simulink model "hydcyl4"  (Simulink 6.0)
settings: Solver=ode45  SolverMode=SingleTasking  StartTime=0.0  StopTime=0.1  FixedStep=0.001  RelTol=1e-5
PreLoadFcn:
  | load newhcd
values from neighbouring files (symbols this model uses):
  Ac = 0.001    [newhcd.mat]
  Beta = 700000000    [newhcd.mat]
  K = 50000    [newhcd.mat]
  Qmax = 0.005    [newhcd.mat]
libraries: hydlib x5
settings Model: Creator=The MathWorks Inc.  LastModifiedBy=batserve  ExtModeTrigMode=oneshot  ExtModeArmWhenConnect=off  ExtModeAutoUpdateStatusClock=off
settings DataIOCC: LimitDataPoints=off  SaveOutput=off  SaveState=on  SignalLoggingName=logsOut
settings OptimizationCC: BooleanDataType=off
settings DebuggingCC: AlgebraicLoopMsg=none  CheckExecutionContextPreStartOutputMsg=on  CheckExecutionContextRuntimeOutputMsg=on  SolverPrmCheckMsg=none  IntegerOverflowMsg=none
settings HardwareCC: TargetUnknown=on

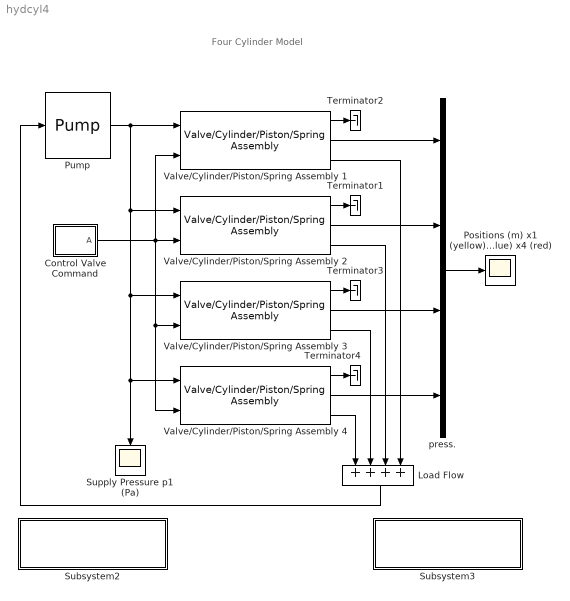
== system hydcyl4 ==
  note: Four Cylinder Model
  Control Valve Command : Subsystem  PropExecContextAcrossSSBoundary=on
      mask Type: Ramp
      mask Display: plot(0,0,100,100,[98,0],[96,0])
  Load Flow : Sum  Orientation=down  Inputs=++++  SaturateOnIntegerOverflow=on  InputSameDT=on
  Positions (m) x1 (yellow) x2 (purple) x3 (blue) x4 (red) : Scope
      settings: TickLabels=on  TimeRange=0.1  YMin=0  YMax=0.019  DataFormat=Array
  Pump : hydlib/Pump  t=[0 0.05 0.051 0.1]  Qpump=Qmax*[1 1 0.5 0.5]  p10=Qmax/C2/2  C2=C2
  Subsystem2 : Subsystem  PropExecContextAcrossSSBoundary=on
      settings: OpenFcn=sim(get_param(0,'CurrentSystem'),0.1)
      mask Type: Button
      mask Display: disp('Double click to run the \nSimulation for 0.1 seconds')
  Subsystem3 : Subsystem  PropExecContextAcrossSSBoundary=on
      settings: OpenFcn=hydrod
      mask Type: Button
      mask Display: disp('Double click for a model\n with two hydraulic cylinders\n  interconnected by a rigid rod')
  Supply Pressure p1 (Pa) : Scope
      settings: Orientation=down  TickLabels=on  TimeRange=0.1  YMin=200000  YMax=1.8e+06  DataFormat=Array
  Terminator{1..4} (4 alike) : Terminator
  Valve/Cylinder/Piston/Spring Assembly 1 : hydlib/Valve//Cylinder//Piston//Spring Assembly  K=K  C1=C1  Ac=Ac  Cd=Cd  rho=rho  V30=V30  beta=Beta
  Valve/Cylinder/Piston/Spring Assembly 2 : hydlib/Valve//Cylinder//Piston//Spring Assembly  K=K/4  C1=C1  Ac=Ac/4  Cd=Cd  rho=rho  V30=V30  beta=Beta
  Valve/Cylinder/Piston/Spring Assembly 3 : hydlib/Valve//Cylinder//Piston//Spring Assembly  K=K*4  C1=C1  Ac=Ac*4  Cd=Cd  rho=rho  V30=V30  beta=Beta
  Valve/Cylinder/Piston/Spring Assembly 4 : hydlib/Valve//Cylinder//Piston//Spring Assembly  K=K  C1=C1  Ac=Ac  Cd=Cd  rho=rho  V30=V30  beta=Beta/1000
  press. : Mux
  wires:
  Valve/Cylinder/Piston/Spring Assembly 4/1 -> Terminator4/1
  Valve/Cylinder/Piston/Spring Assembly 3/1 -> Terminator3/1
  Valve/Cylinder/Piston/Spring Assembly 2/1 -> Terminator1/1
  Valve/Cylinder/Piston/Spring Assembly 1/1 -> Terminator2/1
  Load Flow/1 -> Pump/1
  Valve/Cylinder/Piston/Spring Assembly 1/3 -> Load Flow/4
  Valve/Cylinder/Piston/Spring Assembly 2/3 -> Load Flow/3
  Valve/Cylinder/Piston/Spring Assembly 3/3 -> Load Flow/2
  Valve/Cylinder/Piston/Spring Assembly 4/3 -> Load Flow/1
  Valve/Cylinder/Piston/Spring Assembly 2/2 -> press./2
  Valve/Cylinder/Piston/Spring Assembly 4/2 -> press./4
  Valve/Cylinder/Piston/Spring Assembly 3/2 -> press./3
  Valve/Cylinder/Piston/Spring Assembly 1/2 -> press./1
  Control Valve Command/1(A) -> Valve/Cylinder/Piston/Spring Assembly 3/2, Valve/Cylinder/Piston/Spring Assembly 4/2, Valve/Cylinder/Piston/Spring Assembly 2/2, Valve/Cylinder/Piston/Spring Assembly 1/2
  Pump/1 -> Valve/Cylinder/Piston/Spring Assembly 2/1, Supply Pressure p1 (Pa)/1, Valve/Cylinder/Piston/Spring Assembly 4/1, Valve/Cylinder/Piston/Spring Assembly 3/1, Valve/Cylinder/Piston/Spring Assembly 1/1
  press./1 -> Positions (m) x1 (yellow) x2 (purple) x3 (blue) x4 (red)/1

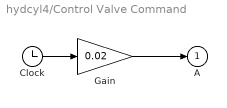
== system hydcyl4/Control Valve Command ==
  Clock : Clock
      settings: Decimation=10
  Gain : Gain  Gain=0.02  SaturateOnIntegerOverflow=on
  A : Outport  InitialOutput=0
  wires:
  Clock/1 -> Gain/1
  Gain/1 -> A/1

== system hydcyl4/Subsystem2 ==

== system hydcyl4/Subsystem3 ==
